simulink model "Lab7_pkt2_2015"  (R2015a)
settings: Solver=ode45  SolverMode=SingleTasking  StartTime=0.0  StopTime=10.0  RelTol=1e-3
values from neighbouring files (symbols this model uses):
  t0 = (k - b)/a    [Lab4.m]    (also in Lab7.m = 71.2)
libraries: cstblocks x2
settings Model: CovMetricSettings=dwe  CovHtmlReporting=off  covSaveCumulativeToWorkspaceVar=off  CovSaveSingleToWorkspaceVar=off  CovExternalEMLEnable=on  Creator=ishiguro  LastModifiedBy=ishiguro
settings DataIOCC: LimitDataPoints=off  SaveFormat=Dataset
settings DebuggingCC: SFUnexpectedBacktrackingDiag=error  SFNoUnconditionalDefaultTransitionDiag=error
settings HardwareCC: ProdBitPerPointer=64  ProdLargestAtomicFloat=Float  ProdIntDivRoundTo=Zero  ProdEndianess=LittleEndian  ProdHWDeviceType=Specified
settings ModelReferenceCC: PropagateSignalLabelsOutOfModel=on
settings GRTTargetCC: TargetLangStandard=C99 (ISO)  GeneratePreprocessorConditionals=Use local settings

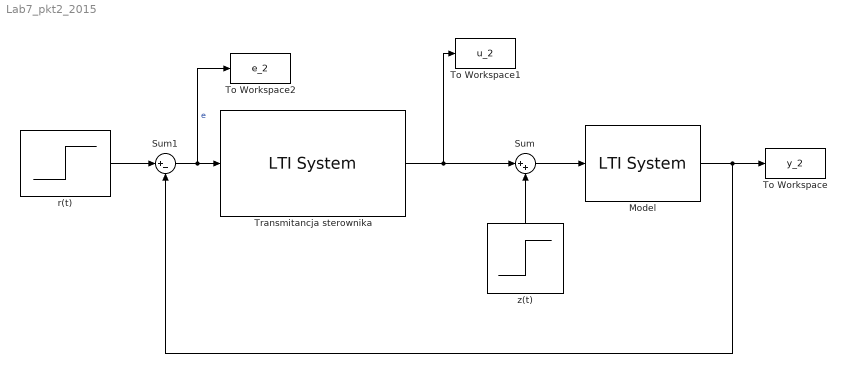
== system Lab7_pkt2_2015 ==
  Model : cstblocks/LTI System  sys=K  IC=[]
  Sum : Sum  Inputs=|++
  Sum1 : Sum  Inputs=|+-
  To Workspace : ToWorkspace  VariableName=y_2  SampleTime=-1
  To Workspace1 : ToWorkspace  VariableName=u_2  SampleTime=-1
  To Workspace2 : ToWorkspace  VariableName=e_2  SampleTime=-1
  Transmitancja sterownika : cstblocks/LTI System  sys=Kr  IC=[]
  r(t) : Step  Time=0  SampleTime=0
  z(t) : Step  Time=t0  SampleTime=0
  wires:
  Sum/1 -> Model/1
  Model/1 -> Sum1/2, To Workspace/1
  z(t)/1 -> Sum/2
  Transmitancja sterownika/1 -> To Workspace1/1, Sum/1
  r(t)/1 -> Sum1/1
  Sum1/1 -> To Workspace2/1, Transmitancja sterownika/1  "e"
